simulink model "StepXYQXF"  (Simulink 5.0)
settings: Solver=ode45  StartTime=0.0  StopTime=6000  RelTol=1e-3
values from neighbouring files (symbols this model uses):
  kd = kp*pi/(4*wr)    [ZieglerDm4_29.m]    (also in Zieglerm4_27.m; example4_15.m = 0.01; example4_16.m = 0.006)
  ki = kp*wr/pi    [ZieglerDm4_29.m]    (also in Zieglerm4_27.m; example4_15.m = 1; example4_16.m = 0.01)
  kp = 0.6*kr    [ZieglerDm4_29.m]    (also in Zieglerm4_27.m; example4_15.m = 1.5; example4_16.m = 1.9)
libraries: simulink_extras x2
settings Model: LastModifiedBy=ThinkPad  ExtModeTrigMode=oneshot  ExtModeArmWhenConnect=off  LimitDataPoints=off  BooleanDataType=off

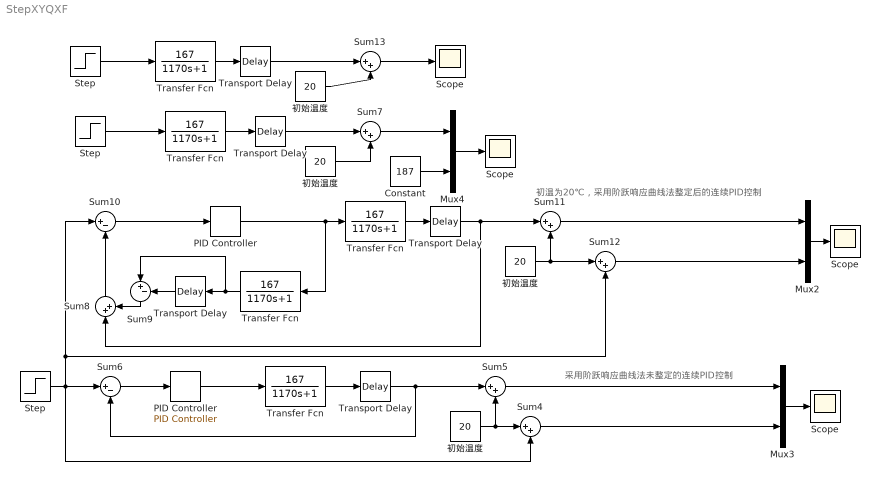
== system StepXYQXF ==
  note: 采用阶跃响应曲线法未整定的连续PID控制
  note: 初温为20℃，采用阶跃响应曲线法整定后的连续PID控制
  "   Transfer Fcn  " : TransferFcn  Numerator=[167]  Denominator=[1170 1]
  " PID Controller " : simulink_extras/Additional Linear/PID Controller  P=kp  I=ki  D=kd
  " Scope" : Scope
      settings: TimeRange=3000  YMin=0  YMax=80  SaveName=StepXYQXFy  DataFormat=Array  MaxDataPoints=500000
  " Scope " : Scope
      settings: TimeRange=2000  YMin=20  YMax=110  SaveName=StepXYQXF  DataFormat=Array  MaxDataPoints=500000
  " Step " : Step  Time=0  After=50  SampleTime=0
  " Transfer Fcn " : TransferFcn  Numerator=[167]  Denominator=[1170 1]
  " Transfer Fcn  " : TransferFcn  Orientation=left  Numerator=[167]  Denominator=[1170 1]
  " Transport Delay " : TransportDelay  Orientation=left  DelayTime=70
  " Transport Delay   " : TransportDelay  DelayTime=70
  " 初始温度 " : Constant  Value=20
  Constant : Constant  Value=187
  Mux2 : Mux  Inputs=2
  Mux3 : Mux  Inputs=2
  Mux4 : Mux  Inputs=2
  "PID Controller " : simulink_extras/Additional Linear/PID Controller  P=0.6  I=0.0003  D=4.5
  "Scope " : Scope
      settings: YMin=0  YMax=80  SaveName=S1  DataFormat=Array  MaxDataPoints=500000
  "Scope  " : Scope
      settings: TimeRange=3000  YMin=0  YMax=80  SaveName=S  DataFormat=Array  MaxDataPoints=500000
  Step : Step  Time=0  SampleTime=0
  "Step " : Step  Time=0  SampleTime=0
  Sum10 : Sum  Inputs=|+-  SaturateOnIntegerOverflow=on
  Sum{4..5,7,11..13} (6 alike) : Sum  Inputs=|++  SaturateOnIntegerOverflow=on
  Sum6 : Sum  Inputs=|+-  SaturateOnIntegerOverflow=on
  Sum8 : Sum  Orientation=up  Inputs=|++  SaturateOnIntegerOverflow=on
  Sum9 : Sum  Orientation=down  Inputs=|+-  SaturateOnIntegerOverflow=on
  Transfer Fcn : TransferFcn  Numerator=[167]  Denominator=[1170 1]
  "Transfer Fcn " : TransferFcn  Numerator=[167]  Denominator=[1170 1]
  "Transport Delay " : TransportDelay  DelayTime=70
  "Transport Delay  " : TransportDelay  DelayTime=70
  "Transport Delay    " : TransportDelay  DelayTime=70
  初始温度 : Constant  Value=20
  "初始温度 " : Constant  Value=20
  "初始温度   " : Constant  Value=20
  wires:
  Transfer Fcn/1 -> "Transport Delay    "/1
  " Step "/1 -> Sum6/1, Sum4/2, Sum10/1, Sum12/2
  "   Transfer Fcn  "/1 -> " Transport Delay   "/1
  " Transport Delay   "/1 -> Sum6/2, Sum5/1
  " PID Controller "/1 -> "   Transfer Fcn  "/1
  Sum6/1 -> " PID Controller "/1
  Mux3/1 -> " Scope "/1
  "Transfer Fcn "/1 -> "Transport Delay  "/1
  "Step "/1 -> "Transfer Fcn "/1
  "Transport Delay  "/1 -> Sum7/1
  " Transfer Fcn "/1 -> "Transport Delay "/1
  "Transport Delay "/1 -> Sum8/1, Sum11/1
  "PID Controller "/1 -> " Transfer Fcn "/1, " Transfer Fcn  "/1
  Sum10/1 -> "PID Controller "/1
  " Transfer Fcn  "/1 -> Sum9/1, " Transport Delay "/1
  " Transport Delay "/1 -> Sum9/2
  Sum8/1 -> Sum10/2
  Mux2/1 -> " Scope"/1
  Sum11/1 -> Mux2/1
  "初始温度 "/1 -> Sum7/2
  初始温度/1 -> Sum11/2, Sum12/1
  Sum9/1 -> Sum8/2
  Sum12/1 -> Mux2/2
  Constant/1 -> Mux4/2
  Sum7/1 -> Mux4/1
  Mux4/1 -> "Scope  "/1
  " 初始温度 "/1 -> Sum4/1, Sum5/2
  Sum5/1 -> Mux3/1
  Sum4/1 -> Mux3/2
  "初始温度   "/1 -> Sum13/2
  "Transport Delay    "/1 -> Sum13/1
  Sum13/1 -> "Scope "/1
  Step/1 -> Transfer Fcn/1
